simulink model "Battery_Management_System"  (R2025b)
settings: Solver=ode1be  StartTime=0.0  StopTime=600  FixedStep=0.1  MaxStep=0.05  RelTol=1e-3  AbsTol=1e-3
PreLoadFcn:
  | Battery_Management_System_param
undefined symbols (not defined in the file): AH, ambient, coolantTemp, iniSOC1, R0_mat, R12, R1_mat, samplingTime, SOC_vec, T_vec, Tau1_mat, V0_mat
libraries: nesl_utility x12, fl_lib x6, ee_lib x2, batteryModule_lib x2
Description:
  | Battery Management System
  | 
  | Copyright 2021-2025 The MathWorks, Inc.
settings Model: Creator=vikrants  LastModifiedBy=smiller
settings SolverCC: AutoScaleAbsTol=off  AlgebraicLoopSolver=TrustRegion
settings DataIOCC: ReturnWorkspaceOutputs=off  SignalLoggingName=logsout_Battery_Pack_Thermal_Management
settings OptimizationCC: ReuseModelBlockBuffer=off
settings DebuggingCC: UnconnectedInputMsg=warning  UnconnectedOutputMsg=warning  UnconnectedLineMsg=warning  SymbolicDimsDataTypeCodeGenerationDiagnostic=none
settings ModelReferenceCC: EnableRefExpFcnMdlSchedulingChecks=on
settings SFSimCC: CustomCodeUndefinedFunction=UseInterfaceOnly
settings RTWCC: GPUComputeCapability=3.5  DLArmComputeVersion=19.05
settings SimscapeCC: SimscapeLogType=all  SimscapeLogSimulationStatistics=on  SimscapeLogName=simlog_Battery_Management_System  SimscapeLogDataHistory=250000.0

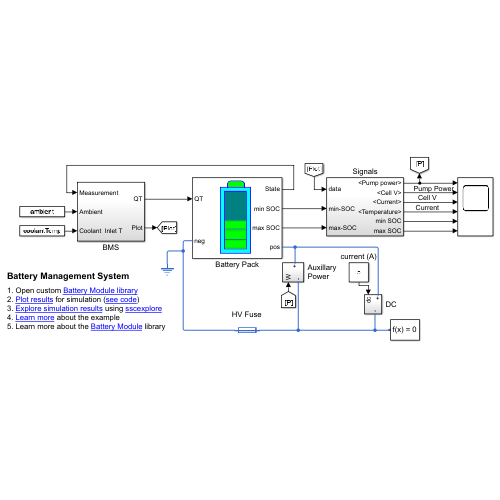
[thumbnail: Simulink's stored preview of the top-level diagram]
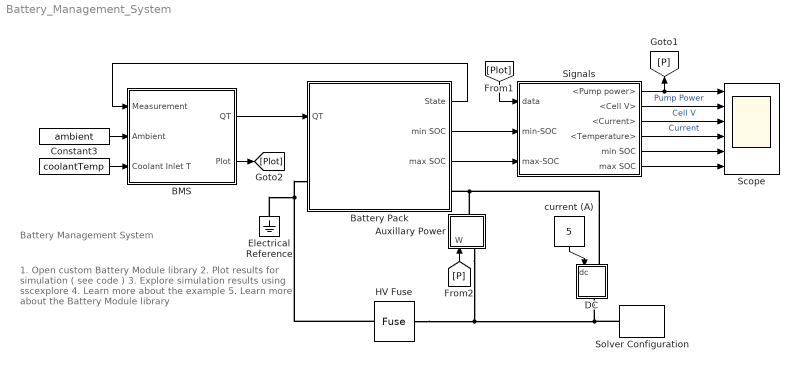
== system Battery_Management_System ==
  note: 1. Open custom Battery Module library
      | 2. Plot results for simulation ( see code )
      | 3. Explore simulation results using sscexplore
      | 4. Learn more about the example
      | 5. Learn more about the Battery Module library
  note: Battery Management System
  " " : Constant  Value=coolantTemp  SampleTime=samplingTime
  Auxillary Power : Subsystem
  BMS : Subsystem
  Battery Pack : Subsystem
      mask Display: image('Battery_Management_System_icon.png'); % Use "Edit Image" on toolstrip to change.
  Constant3 : Constant  Value=ambient  SampleTime=samplingTime
  DC : Subsystem
  Electrical Reference : fl_lib/Electrical/Electrical Elements/Electrical Reference
  HV Fuse : ee_lib/Switches & Breakers/Fuse  prm=1  I_rated=100 A  melt_margin=4  T_fuse=0 s  I2t=1 s*A^2  I_vec=[1.9, 2, 2.5, 30] A  t_vec=[10000, 1, .3, .001] s  R_closed=0.0005 Ohm  G_open=1e-8 1/Ohm  exposemeasurement=ee.enum.exposemeasurement.hidden
      settings: InternalSimscapePortConfiguration="{\"Bottom\":[],\"Left\":[{\"id\":\"p\",\"label\":\"\",\"type\":\"foundation.electrical.electrical\"}],\"Right\":[{\"id\":\"n\",\"label\":\"\",\"type\":\"foundation.electrical.electrical\"}],\"Top\":[]}"
  Scope : Scope  NumInputPorts=6
      settings: ActiveDisplayYMinimum=-15.625  ActiveDisplayYMaximum=140.625  DataLoggingVariableName=Battery_Management_System_Scope
  Signals : Subsystem
  Solver Configuration : nesl_utility/Solver Configuration  PhysicalDomain=network_engine_domain  SubClassName=solver  LeftPortType=input  RightPortType=generic  Tones=[]  Harmonics=[]  SimulateNoise=off  Profile=off  UseLocalSampling=off  EnableSwitchedLinearOptims=on  FrequencyDomain=off  UseCCode=off  RelTol=0.001  AbsTol=1e-06  MinStep=1e-09  ToWorkspace=off  RevertToSquareIcSolve=off  NumHomotopyIterations=100  PhasorMode=off  PhasorModeNumHarmonics=1  ConsistencySolver=NEWTON_FTOL  IndexReductionMethod=DerivativeReplacement  DoDC=off  ResidualTolerance=1e-09  ConsistencyTolSource=GLOBAL  ConsistencyAbsTol=0.001  ConsistencyRelTol=0.001  ConsistencyTolFactor=0.001  UseLocalSolver=on  LocalSolverChoice=NE_BACKWARD_EULER_ADVANCER  ResolveIndetEquations=on  FunctionEvalNumThread=1  LocalSolverSampleTime=0.1  DoFixedCost=on  MaxNonlinIter=3  MaxModeIter=2  ComputeImpulses=off  ImpulseIterations=2  LinearAlgebra=auto  LinearAlgebraNumThread=0  EquationFormulation=NE_TIME_EF  DelaysMemoryBudget=1024  AutomaticFiltering=on  FilteringTimeConstant=0.001  PartitionStorageMethod=AS_NEEDED  PartitionMemoryBudget=1024  PartitionMethod=ROBUST  MultibodyUseLocalSolver=off  MultibodyLocalSolverChoice=ODE1  MultibodyLocalSolverSampleTime=0.001
  current (A) : Constant  Value=5
  wires:
  Battery Pack/1(State) -> BMS/1(Measurement)
  Constant3/1 -> BMS/2(Ambient)
  " "/1 -> BMS/3(Coolant Inlet T)
  BMS/1(QT) -> Battery Pack/1(QT)
  BMS/2(Plot) -> [Plot]
  [P] -> Auxillary Power/1(W)
  current (A)/1 -> DC/1(dc)
  Battery Pack/3(max SOC) -> Signals/3(max-SOC)
  Signals/1(<Pump power>) -> Scope/1, [P]  "Pump Power"
  [Plot] -> Signals/1(data)
  Battery Pack/2(min SOC) -> Signals/2(min-SOC)
  Signals/2(<Cell V>) -> Scope/2  "Cell V"
  Signals/3(<Current>) -> Scope/3  "Current"
  Signals/4(<Temperature>) -> Scope/4
  Signals/5(min SOC) -> Scope/5
  Signals/6(max SOC) -> Scope/6
  connections:
  Auxillary Power/LConn1 -- HV Fuse/LConn1 -- Solver Configuration/RConn1 -- DC/RConn1
  Auxillary Power/RConn1 -- Battery Pack/RConn1 -- DC/LConn1
  HV Fuse/RConn1 -- Electrical Reference/LConn1 -- Battery Pack/LConn1

== system Battery_Management_System/Auxillary Power ==
  W : Inport
  Aux. Power : ee_lib/Passive/Dynamic Load  load_type=ee.enum.dc_ac.dc  min_supply_voltage=20 V  pow_min=1e-3 W  G_reverse=1e-6 S  deltaV=1e-3 V  f0=60 Hz  Vrms_min=200 V  tau=0.01 s  Vrms_ini=300 V  Vang_ini=0 deg
      settings: InternalSimscapePortConfiguration="{\"Bottom\":[],\"Left\":[{\"id\":\"p\",\"label\":\"+\",\"type\":\"foundation.electrical.electrical\"}],\"Right\":[{\"id\":\"n\",\"label\":\"-\",\"type\":\"foundation.electrical.electrical\"}],\"Top\":[{\"id\":\"P\",\"label\":\"P\",\"type\":\"input\"}]}"
  P : nesl_utility/Simulink-PS Converter  PhysicalDomain=network_engine_domain  SubClassName=ps_input  LeftPortType=input  RightPortType=output  PseudoPeriodic=off  Frequencies=[]  NoiseDistribution=none  NoiseParameters=[]  Unit=J/s  AffineConversion=off  FilteringAndDerivatives=provide  SimscapeFilterOrder=1  InputFilterTimeConstant=0.001  UdotUserProvided=0
  + : PMIOPort  Side=Right
  - : PMIOPort  Port=2  Side=Left
  wires:
  W/1 -> P/1
  connections:
  P/RConn1 -- Aux. Power/LConn2
  Aux. Power/LConn1 -- -/RConn1
  Aux. Power/RConn1 -- +/RConn1

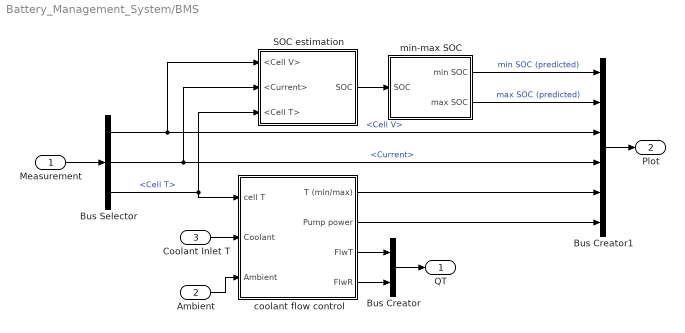
== system Battery_Management_System/BMS ==
  Measurement : Inport
  Ambient : Inport  Port=2  Unit=K
  Coolant Inlet T : Inport  Port=3  Unit=K
  Bus Creator : BusCreator  Inputs=2
  Bus Creator1 : BusCreator  Inputs=6
  Bus Selector : BusSelector  OutputSignals=Cell V,Current,Cell T
  SOC estimation : Subsystem
  coolant flow control : Subsystem
  min-max SOC : Subsystem
  QT : Outport
  Plot : Outport  Port=2
  wires:
  Bus Creator/1 -> QT/1
  Measurement/1 -> Bus Selector/1
  Bus Creator1/1 -> Plot/1
  Bus Selector/1 -> SOC estimation/1(<Cell V>), Bus Creator1/3  "<Cell V>"
  Bus Selector/3 -> SOC estimation/3(<Cell T>), coolant flow control/1(cell T)  "<Cell T>"
  Bus Selector/2 -> Bus Creator1/4, SOC estimation/2(<Current>)  "<Current>"
  SOC estimation/1(SOC) -> min-max SOC/1(SOC)
  min-max SOC/1(min SOC) -> Bus Creator1/1  "min SOC (predicted)"
  min-max SOC/2(max SOC) -> Bus Creator1/2  "max SOC (predicted)"
  Coolant Inlet T/1 -> coolant flow control/2(Coolant)
  Ambient/1 -> coolant flow control/3(Ambient)
  coolant flow control/3(FlwT) -> Bus Creator/1
  coolant flow control/4(FlwR) -> Bus Creator/2
  coolant flow control/2(Pump power) -> Bus Creator1/6
  coolant flow control/1(T (min/max)) -> Bus Creator1/5

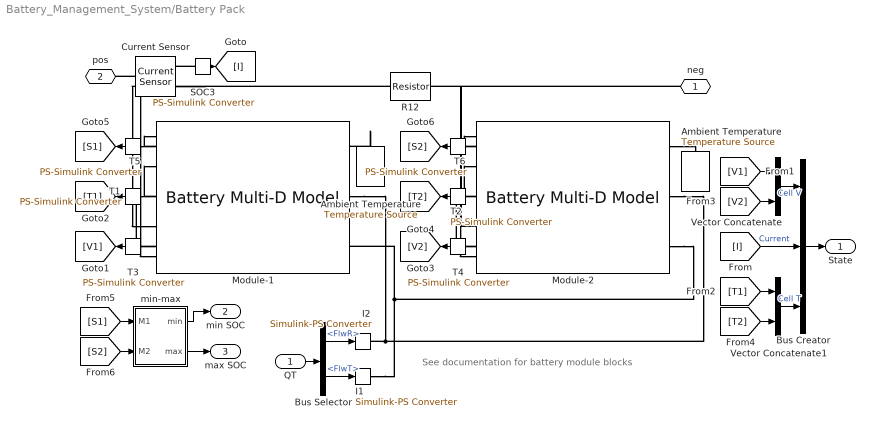
== system Battery_Management_System/Battery Pack ==
  note: See documentation for battery module blocks
  QT : Inport
  Ambient Temperature : fl_lib/Thermal/Thermal Sources/Temperature Source  temperature=ambient K
  "Ambient Temperature " : fl_lib/Thermal/Thermal Sources/Temperature Source  temperature=ambient K
  Bus Creator : BusCreator  Inputs=3
  Bus Selector : BusSelector  OutputSignals=FlwR,FlwT
  Current Sensor : fl_lib/Electrical/Electrical Sensors/Current Sensor
  I1 : nesl_utility/Simulink-PS Converter  PhysicalDomain=network_engine_domain  SubClassName=ps_input  LeftPortType=input  RightPortType=output  PseudoPeriodic=off  Frequencies=[]  NoiseDistribution=none  NoiseParameters=[]  Unit=K  AffineConversion=off  FilteringAndDerivatives=provide  SimscapeFilterOrder=1  InputFilterTimeConstant=0.001  UdotUserProvided=0
  I2 : nesl_utility/Simulink-PS Converter  PhysicalDomain=network_engine_domain  SubClassName=ps_input  LeftPortType=input  RightPortType=output  PseudoPeriodic=off  Frequencies=[]  NoiseDistribution=none  NoiseParameters=[]  Unit=1  AffineConversion=off  FilteringAndDerivatives=provide  SimscapeFilterOrder=1  InputFilterTimeConstant=0.001  UdotUserProvided=0
  Module-1 : batteryModule_lib/Battery Multi-D Model  modelComplexity=batteryModule.batteryAbstractionLevel.detailed  LUTpointsTemp=T_vec K  cellAH=AH A*hr  LUTpointsSOC=SOC_vec  V0_mat=V0_mat V  prm_dir=simscape.enum.tablebattery.prm_dir.noCurrentDirectionality  R0_mat=R0_mat Ohm  R0_dis_mat=[.03, .015, .002; .04, .017, .008; .039, .012, .006; .027, .013, .021] Ohm  R0_ch_mat=[.03, .015, .002; .04, .017, .008; .039, .012, .006; .027, .013, .021] Ohm  prm_leak=simscape.enum.tablebattery.prm_leak.disabled  Rleak_vec=[8000, 7000, 6000] Ohm  extrapolation_option=simscape.enum.extrapolation.linear  prm_dyn=simscape.enum.tablebattery.prm_dyn.rc1  R1_mat=R1_mat Ohm  tau1_mat=Tau1_mat s  R2_mat=R2_mat Ohm  tau2_mat=Tau2_mat s  R3_mat=[.014, .382, .407; .028, .006, .007; .014, .007, .006; .333, .956, .912] Ohm  tau3_mat=[1, 44, 5644; 11, 24, 506; 2, 14, 330; 3310, 13419, 30216] s  R4_mat=[.014, .382, .407; .028, .006, .007; .014, .007, .006; .333, .956, .912] Ohm  tau4_mat=[1, 44, 5644; 11, 24, 506; 2, 14, 330; 3310, 13419, 30216] s  R5_mat=[.014, .382, .407; .028, .006, .007; .014, .007, .006; .333, .956, .912] Ohm  tau5_mat=[1, 44, 5644; 11, 24, 506; 2, 14, 330; 3310, 13419, 30216] s  prm_fade=simscape.enum.tablebattery.prm_fade.equations  N0=Ndisc  dV0=delV0  dR0=delR0  dAH=delAH0  dRleak=0  dR1=delR1  dR2=delR2  dR3=0  dR4=0  dR5=0  N0vec=[100, 200, 300]  Tfadevec=[298.15, 323.15] K  dV0vec=[0, 0, 0]  dR0vec=[0, 0, 0]  dAHvec=[0, 0, 0]  dRleakvec=[0, 0, 0]  dR1vec=[0, 0, 0]  dR2vec=[0, 0, 0]  dR3vec=[0, 0, 0]  dR4vec=[0, 0, 0]  dR5vec=[0, 0, 0]  dV0mat=[0, 0; 0, 0; 0, 0]  dR0mat=[0, 0; 0, 0; 0, 0]  dAHmat=[0, 0; 0, 0; 0, 0]  dRleakmat=[0, 0; 0, 0; 0, 0]  dR1mat=[0, 0; 0, 0; 0, 0]  dR2mat=[0, 0; 0, 0; 0, 0]  dR3mat=[0, 0; 0, 0; 0, 0]  dR4mat=[0, 0; 0, 0; 0, 0]  dR5mat=[0, 0; 0, 0; 0, 0]  cellThermalMass=MdotCp J/K  cellThermalCond=K_cell W/(m*K)  cellThermalCond_inPlane=20 W/(m*K)  Ns=Ns1  Np=Np1  cellTypeSelection=batteryModule.batteryTypeSelection.pouch  cellHeight=cell_H m  cellWidth=cell_W m  cellThickness=cell_T m  cellDiameter=0.018 m  cellCylinLine=3  moduleExternalR=Rext1 Ohm  moduleCellBalancing=batteryModule.batteryCellBalancing.none  passiveShuntR=50 Ohm  passiveSWclosedR=0.01 Ohm  passiveSWopenCond=1e-8 1/Ohm  passiveSWthreshold=0.5  moduleCellVoltages=batteryModule.batteryCellVoltages.yes  thermalManagement=batteryModule.batteryCoolingSystem.thermalPort  cellHeatTrCoeff=h_cell W/(m^2 * K)  thermal_moduleBottom=batteryModule.batteryThermalPortSelection.thermalLUT  htc_bottom=1 W/(m^2 * K)  moduleCooling_b=Q1 W/K  LUTpointsFlowrate_b=Flowrate_vec kg/s  LUTpointsTemp_b=T_vec K  thermal_moduleTop=batteryModule.batteryThermalPortSelection.convectionBC  htc_top=h_cell W/(m^2 * K)  moduleCooling_t=zeros(3, 6, 10) W/K  LUTpointsFlowrate_t=[.01, .02, .03, .04, .05, .06] kg/s  LUTpointsTemp_t=[273.15, 298.15, 323.15] K  thermal_moduleRight=batteryModule.batteryThermalPortSelection.convectionBC  htc_right=h_cell W/(m^2 * K)  moduleCooling_r=zeros(3, 6, 10) W/K  LUTpointsFlowrate_r=[.01, .02, .03, .04, .05, .06] kg/s  LUTpointsTemp_r=[273.15, 298.15, 323.15] K  thermal_moduleLeft=batteryModule.batteryThermalPortSelection.convectionBC  htc_left=h_cell W/(m^2 * K)  moduleCooling_l=zeros(3, 6, 10) W/K  LUTpointsFlowrate_l=[.01, .02, .03, .04, .05, .06] kg/s  LUTpointsTemp_l=[273.15, 298.15, 323.15] K  thermal_modulePos=batteryModule.batteryThermalPortSelection.convectionBC  htc_pos=h_cell W/(m^2 * K)  moduleCooling_p=zeros(3, 6, 10) W/K  LUTpointsFlowrate_p=[.01, .02, .03, .04, .05, .06] kg/s  LUTpointsTemp_p=[273.15, 298.15, 323.15] K  thermal_moduleNeg=batteryModule.batteryThermalPortSelection.convectionBC  htc_neg=h_cell W/(m^2 * K)  moduleCooling_n=zeros(3, 6, 10) W/K  LUTpointsFlowrate_n=[.01, .02, .03, .04, .05, .06] kg/s  LUTpointsTemp_n=[273.15, 298.15, 323.15] K  moduleExtHeat=extQ1 W  cellTemp=iniT1 K  cellSOC=iniSOC1  moduleCellAHpercentVar=iniAH1  moduleCellLeakPercentVar=ones(1, 10)  moduleCellR0PercentVar=iniR01
      settings: InternalSimscapePortConfiguration="{\"Bottom\":[],\"Left\":[{\"id\":\"outputCellSOC\",\"label\":\"SOC\",\"type\":\"output\"},{\"id\":\"outputCellTemp\",\"label\":\"Temp\",\"type\":\"output\"},{\"id\":\"outputCellV\",\"label\":\"V\",\"type\":\"output\"}],\"Right\":[{\"id\":\"H\",\"label\":\"Amb\",\"type\":\"foundation.thermal.thermal\"},{\"id\":\"frac_b\",\"label\":\"FlwR\",\"type\":\"input\"},{\"id\":\"delT_b\",\"label\":\"FlwT\",\"type\":\"input\"}],\"Top\":[{\"id\":\"p\",\"label\":\"pos\",\"type\":\"foundation.electrical.electrical\"},{\"id\":\"n\",\"label\":\"neg\",\"type\":\"foundation.electrical.electrical\"}]}"
  Module-2 : batteryModule_lib/Battery Multi-D Model  modelComplexity=batteryModule.batteryAbstractionLevel.detailed  LUTpointsTemp=T_vec K  cellAH=AH A*hr  LUTpointsSOC=SOC_vec  V0_mat=V0_mat V  prm_dir=simscape.enum.tablebattery.prm_dir.noCurrentDirectionality  R0_mat=R0_mat Ohm  R0_dis_mat=[.03, .015, .002; .04, .017, .008; .039, .012, .006; .027, .013, .021] Ohm  R0_ch_mat=[.03, .015, .002; .04, .017, .008; .039, .012, .006; .027, .013, .021] Ohm  prm_leak=simscape.enum.tablebattery.prm_leak.disabled  Rleak_vec=[8000, 7000, 6000] Ohm  extrapolation_option=simscape.enum.extrapolation.linear  prm_dyn=simscape.enum.tablebattery.prm_dyn.rc1  R1_mat=R1_mat Ohm  tau1_mat=Tau1_mat s  R2_mat=R2_mat Ohm  tau2_mat=Tau2_mat s  R3_mat=[.014, .382, .407; .028, .006, .007; .014, .007, .006; .333, .956, .912] Ohm  tau3_mat=[1, 44, 5644; 11, 24, 506; 2, 14, 330; 3310, 13419, 30216] s  R4_mat=[.014, .382, .407; .028, .006, .007; .014, .007, .006; .333, .956, .912] Ohm  tau4_mat=[1, 44, 5644; 11, 24, 506; 2, 14, 330; 3310, 13419, 30216] s  R5_mat=[.014, .382, .407; .028, .006, .007; .014, .007, .006; .333, .956, .912] Ohm  tau5_mat=[1, 44, 5644; 11, 24, 506; 2, 14, 330; 3310, 13419, 30216] s  prm_fade=simscape.enum.tablebattery.prm_fade.equations  N0=Ndisc  dV0=delV0  dR0=delR0  dAH=delAH0  dRleak=0  dR1=delR1  dR2=delR2  dR3=0  dR4=0  dR5=0  N0vec=[100, 200, 300]  Tfadevec=[298.15, 323.15] K  dV0vec=[0, 0, 0]  dR0vec=[0, 0, 0]  dAHvec=[0, 0, 0]  dRleakvec=[0, 0, 0]  dR1vec=[0, 0, 0]  dR2vec=[0, 0, 0]  dR3vec=[0, 0, 0]  dR4vec=[0, 0, 0]  dR5vec=[0, 0, 0]  dV0mat=[0, 0; 0, 0; 0, 0]  dR0mat=[0, 0; 0, 0; 0, 0]  dAHmat=[0, 0; 0, 0; 0, 0]  dRleakmat=[0, 0; 0, 0; 0, 0]  dR1mat=[0, 0; 0, 0; 0, 0]  dR2mat=[0, 0; 0, 0; 0, 0]  dR3mat=[0, 0; 0, 0; 0, 0]  dR4mat=[0, 0; 0, 0; 0, 0]  dR5mat=[0, 0; 0, 0; 0, 0]  cellThermalMass=MdotCp J/K  cellThermalCond=K_cell W/(m*K)  cellThermalCond_inPlane=20 W/(m*K)  Ns=Ns2  Np=Np2  cellTypeSelection=batteryModule.batteryTypeSelection.pouch  cellHeight=cell_H m  cellWidth=cell_W m  cellThickness=cell_T m  cellDiameter=0.018 m  cellCylinLine=3  moduleExternalR=Rext2 Ohm  moduleCellBalancing=batteryModule.batteryCellBalancing.none  passiveShuntR=50 Ohm  passiveSWclosedR=0.01 Ohm  passiveSWopenCond=1e-8 1/Ohm  passiveSWthreshold=0.5  moduleCellVoltages=batteryModule.batteryCellVoltages.yes  thermalManagement=batteryModule.batteryCoolingSystem.thermalPort  cellHeatTrCoeff=h_cell W/(m^2 * K)  thermal_moduleBottom=batteryModule.batteryThermalPortSelection.thermalLUT  htc_bottom=1 W/(m^2 * K)  moduleCooling_b=Q2 W/K  LUTpointsFlowrate_b=Flowrate_vec kg/s  LUTpointsTemp_b=T_vec K  thermal_moduleTop=batteryModule.batteryThermalPortSelection.convectionBC  htc_top=h_cell W/(m^2 * K)  moduleCooling_t=zeros(3, 6, 10) W/K  LUTpointsFlowrate_t=[.01, .02, .03, .04, .05, .06] kg/s  LUTpointsTemp_t=[273.15, 298.15, 323.15] K  thermal_moduleRight=batteryModule.batteryThermalPortSelection.convectionBC  htc_right=h_cell W/(m^2 * K)  moduleCooling_r=zeros(3, 6, 10) W/K  LUTpointsFlowrate_r=[.01, .02, .03, .04, .05, .06] kg/s  LUTpointsTemp_r=[273.15, 298.15, 323.15] K  thermal_moduleLeft=batteryModule.batteryThermalPortSelection.convectionBC  htc_left=h_cell W/(m^2 * K)  moduleCooling_l=zeros(3, 6, 10) W/K  LUTpointsFlowrate_l=[.01, .02, .03, .04, .05, .06] kg/s  LUTpointsTemp_l=[273.15, 298.15, 323.15] K  thermal_modulePos=batteryModule.batteryThermalPortSelection.convectionBC  htc_pos=h_cell W/(m^2 * K)  moduleCooling_p=zeros(3, 6, 10) W/K  LUTpointsFlowrate_p=[.01, .02, .03, .04, .05, .06] kg/s  LUTpointsTemp_p=[273.15, 298.15, 323.15] K  thermal_moduleNeg=batteryModule.batteryThermalPortSelection.convectionBC  htc_neg=h_cell W/(m^2 * K)  moduleCooling_n=zeros(3, 6, 10) W/K  LUTpointsFlowrate_n=[.01, .02, .03, .04, .05, .06] kg/s  LUTpointsTemp_n=[273.15, 298.15, 323.15] K  moduleExtHeat=extQ2 W  cellTemp=iniT2 K  cellSOC=iniSOC2  moduleCellAHpercentVar=iniAH2  moduleCellLeakPercentVar=ones(1, 10)  moduleCellR0PercentVar=iniR02
      settings: InternalSimscapePortConfiguration="{\"Bottom\":[],\"Left\":[{\"id\":\"outputCellSOC\",\"label\":\"SOC\",\"type\":\"output\"},{\"id\":\"outputCellTemp\",\"label\":\"Temp\",\"type\":\"output\"},{\"id\":\"outputCellV\",\"label\":\"V\",\"type\":\"output\"}],\"Right\":[{\"id\":\"H\",\"label\":\"Amb\",\"type\":\"foundation.thermal.thermal\"},{\"id\":\"frac_b\",\"label\":\"FlwR\",\"type\":\"input\"},{\"id\":\"delT_b\",\"label\":\"FlwT\",\"type\":\"input\"}],\"Top\":[{\"id\":\"p\",\"label\":\"pos\",\"type\":\"foundation.electrical.electrical\"},{\"id\":\"n\",\"label\":\"neg\",\"type\":\"foundation.electrical.electrical\"}]}"
  R12 : fl_lib/Electrical/Electrical Elements/Resistor  R=R12 Ohm  i_specify=off  i_priority=None  i=0 A  i_nominal_specify=off  i_nominal_value=1  i_nominal_unit=A  v_specify=off  v_priority=None  v=0 V  v_nominal_specify=off  v_nominal_value=1  v_nominal_unit=V
  SOC3 : nesl_utility/PS-Simulink Converter  PhysicalDomain=network_engine_domain  SubClassName=ps_output  LeftPortType=input  RightPortType=output  PseudoPeriodic=off  Frequencies=[]  VectorFormat=1-D array  Unit=inherit  AffineConversion=off
  T{1..6} (6 alike) : nesl_utility/PS-Simulink Converter  PhysicalDomain=network_engine_domain  SubClassName=ps_output  LeftPortType=input  RightPortType=output  PseudoPeriodic=off  Frequencies=[]  VectorFormat=1-D array  Unit=inherit  AffineConversion=off
  Vector Concatenate : Concatenate
  Vector Concatenate1 : Concatenate
  min-max : Subsystem
  neg : PMIOPort  Side=Left
  pos : PMIOPort  Port=2  Side=Right
  State : Outport
  min SOC : Outport  Port=2
  max SOC : Outport  Port=3
  wires:
  Bus Creator/1 -> State/1
  Vector Concatenate/1 -> Bus Creator/1  "Cell V"
  SOC3/1 -> [I]
  [V1] -> Vector Concatenate/1
  T3/1 -> [V1]
  [T1] -> Vector Concatenate1/1
  T2/1 -> [T2]
  T4/1 -> [V2]
  T1/1 -> [T1]
  [T2] -> Vector Concatenate1/2
  [V2] -> Vector Concatenate/2
  Vector Concatenate1/1 -> Bus Creator/3  "Cell T"
  [I] -> Bus Creator/2  "Current"
  QT/1 -> Bus Selector/1
  Bus Selector/1 -> I2/1  "<FlwR>"
  Bus Selector/2 -> I1/1  "<FlwT>"
  T5/1 -> [S1]
  T6/1 -> [S2]
  min-max/1(min) -> min SOC/1
  min-max/2(max) -> max SOC/1
  [S1] -> min-max/1(M1)
  [S2] -> min-max/2(M2)
  connections:
  T1/LConn1 -- Module-1/LConn2
  R12/LConn1 -- Module-1/LConn5
  T2/LConn1 -- Module-2/LConn2
  Module-2/LConn4 -- R12/RConn1
  neg/RConn1 -- Module-2/LConn5
  T3/LConn1 -- Module-1/LConn3
  T4/LConn1 -- Module-2/LConn3
  Current Sensor/LConn1 -- pos/RConn1
  Current Sensor/RConn2 -- Module-1/LConn4
  SOC3/LConn1 -- Current Sensor/RConn1
  Ambient Temperature/LConn1 -- Module-1/RConn1
  Module-2/RConn1 -- "Ambient Temperature "/LConn1
  Module-1/RConn2 -- Module-2/RConn2 -- I2/RConn1
  I1/RConn1 -- Module-2/RConn3 -- Module-1/RConn3
  T5/LConn1 -- Module-1/LConn1
  T6/LConn1 -- Module-2/LConn1

== system Battery_Management_System/DC ==
  dc : Inport
  Current Source : fl_lib/Electrical/Electrical Sources/Controlled Current Source
  Gain : Gain  Gain=-1
  I : nesl_utility/Simulink-PS Converter  PhysicalDomain=network_engine_domain  SubClassName=ps_input  LeftPortType=input  RightPortType=output  PseudoPeriodic=off  Frequencies=[]  NoiseDistribution=none  NoiseParameters=[]  Unit=A  AffineConversion=off  FilteringAndDerivatives=provide  SimscapeFilterOrder=1  InputFilterTimeConstant=0.001  UdotUserProvided=0
  + : PMIOPort  Side=Left
  - : PMIOPort  Port=2  Side=Right
  wires:
  Gain/1 -> I/1
  dc/1 -> Gain/1
  connections:
  I/RConn1 -- Current Source/RConn1
  Current Source/LConn1 -- +/RConn1
  Current Source/RConn2 -- -/RConn1

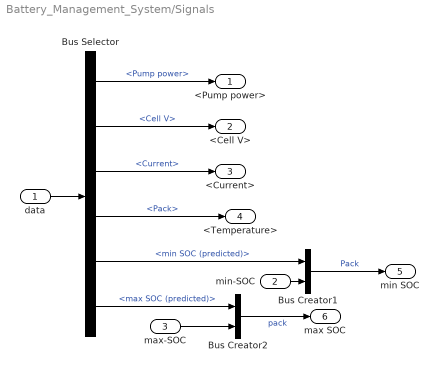
== system Battery_Management_System/Signals ==
  data : Inport
  min-SOC : Inport  Port=2
  max-SOC : Inport  Port=3
  Bus Creator1 : BusCreator  Inputs=2
  Bus Creator2 : BusCreator  Inputs=2
  Bus Selector : BusSelector  OutputSignals=Pump power,Cell V,Current,Pack,min SOC (predicted),max SOC (predicted)
  <Pump power> : Outport
  <Cell V> : Outport  Port=2
  <Current> : Outport  Port=3
  <Temperature> : Outport  Port=4
  min SOC : Outport  Port=5
  max SOC : Outport  Port=6
  wires:
  min-SOC/1 -> Bus Creator1/2
  Bus Creator2/1 -> max SOC/1  "pack"
  Bus Selector/2 -> <Cell V>/1  "<Cell V>"
  Bus Creator1/1 -> min SOC/1  "Pack"
  max-SOC/1 -> Bus Creator2/2
  Bus Selector/4 -> <Temperature>/1  "<Pack>"
  data/1 -> Bus Selector/1
  Bus Selector/5 -> Bus Creator1/1  "<min SOC (predicted)>"
  Bus Selector/3 -> <Current>/1  "<Current>"
  Bus Selector/1 -> <Pump power>/1  "<Pump power>"
  Bus Selector/6 -> Bus Creator2/1  "<max SOC (predicted)>"

== system Battery_Management_System/BMS/SOC estimation ==
  <Cell V> : Inport
  <Current> : Inport  Port=2
  <Cell T> : Inport  Port=3
  AEKF 1TC : Subsystem  TreatAsAtomicUnit=on
  SeriesStringData <Ns=20,Np=1> : MATLAB Function  TreatAsAtomicUnit=on
  SOC : Outport
  wires:
  SeriesStringData <Ns=20,Np=1>/1(Is) -> AEKF 1TC/1(Current)
  <Cell V>/1 -> SeriesStringData <Ns=20,Np=1>/3(V)
  AEKF 1TC/1(SOC) -> SOC/1
  SeriesStringData <Ns=20,Np=1>/3(Vs) -> AEKF 1TC/3(Voltage)
  <Current>/1 -> SeriesStringData <Ns=20,Np=1>/1(I)
  SeriesStringData <Ns=20,Np=1>/2(Ts) -> AEKF 1TC/2(Temperature)
  <Cell T>/1 -> SeriesStringData <Ns=20,Np=1>/2(T)

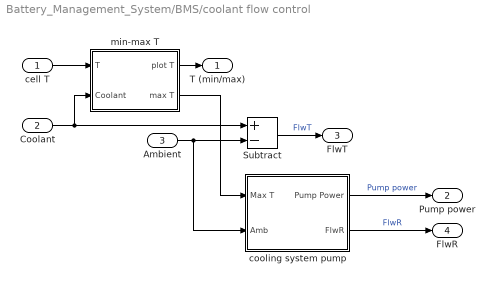
== system Battery_Management_System/BMS/coolant flow control ==
  cell T : Inport
  Coolant : Inport  Port=2
  Ambient : Inport  Port=3
  Subtract : Sum  Inputs=+-
  cooling system pump : Subsystem
  min-max T : Subsystem
  T (min/max) : Outport
  Pump power : Outport  Port=2
  FlwT : Outport  Port=3
  FlwR : Outport  Port=4
  wires:
  cell T/1 -> min-max T/1(T)
  min-max T/2(max T) -> cooling system pump/1(Max T)
  Coolant/1 -> min-max T/2(Coolant), Subtract/1
  cooling system pump/2(FlwR) -> FlwR/1  "FlwR"
  cooling system pump/1(Pump Power) -> Pump power/1  "Pump power"
  Subtract/1 -> FlwT/1  "FlwT"
  min-max T/1(plot T) -> T (min/max)/1
  Ambient/1 -> cooling system pump/2(Amb), Subtract/2

== system Battery_Management_System/BMS/min-max SOC ==
  SOC : Inport
  MinMax2 : MinMax
  MinMax3 : MinMax  Function=max
  min SOC : Outport
  max SOC : Outport  Port=2
  wires:
  MinMax3/1 -> max SOC/1
  SOC/1 -> MinMax2/1, MinMax3/1
  MinMax2/1 -> min SOC/1

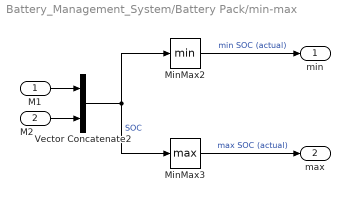
== system Battery_Management_System/Battery Pack/min-max ==
  M1 : Inport
  M2 : Inport  Port=2
  MinMax2 : MinMax
  MinMax3 : MinMax  Function=max
  Vector Concatenate2 : Concatenate
  min : Outport
  max : Outport  Port=2
  wires:
  MinMax3/1 -> max/1  "max SOC (actual)"
  MinMax2/1 -> min/1  "min SOC (actual)"
  Vector Concatenate2/1 -> MinMax3/1, MinMax2/1  "SOC"
  M1/1 -> Vector Concatenate2/1
  M2/1 -> Vector Concatenate2/2

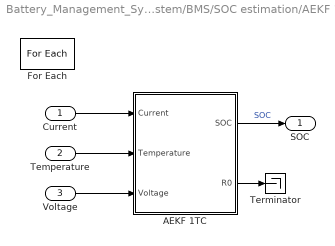
== system Battery_Management_System/BMS/SOC estimation/AEKF 1TC ==
  Current : Inport  Partition=on  PartitionDimension=1  PartitionWidth=1  PartitionOffset=0
  Temperature : Inport  Port=2  Partition=on  PartitionDimension=1  PartitionWidth=1  PartitionOffset=0
  Voltage : Inport  Port=3  Partition=on  PartitionDimension=1  PartitionWidth=1  PartitionOffset=0
  AEKF 1TC : Subsystem  mask(Adaptive Extended Kalman Filter SOC estimator){SOC_vec=SOC_vec, T_vec=T_vec, R0_mat=R0_mat, R1_mat=R1_mat, tau1_mat=Tau1_mat, V0_mat=V0_mat, AH=AH, Reol=0.05, Ts=1, Q=1e-8*eye(3), R=1e-2, P0=[1e-5 0 0; 0 1 0; 0 0 0.0125], x0=[iniSOC1(1);0;9.4e-3]}
      mask prompts: SOC_vec "Vector of state-of-charge values, SOC"; T_vec "Vector of temperatures, T"; R0_mat "Terminal resistance, R0(SOC,T)"; R1_mat "First polarization resistance, R1(SOC,T)"; tau1_mat "First time constant, tau1(SOC,T)"; V0_mat "No-load voltage, V0(SOC,T)"; AH "Ampere-hour rating"; Reol "End of life resistance"; Ts "Sample time"; Q "Covariance of the process noise, Q"; R "Covariance matrix of the measurement noise, R"; P0 "Initial state error covariance, P0"; x0 "Initial state"
      mask help: This block implements an Adaptive Extended Kalman Filter battery SOC estimator based on a one time constant battery model.
      mask init:
      | C1_mat=tau1_mat./R1_mat;
      | 
      | dV0_mat=zeros(size(V0_mat));
      | [n_soc,m_soc]=size(SOC_vec);
      | if n_soc<m_soc
      |     dV0_mat(2:end,:)=diff(V0_mat,1,1)./diff(SOC_vec');
      | else
      |     dV0_mat(2:end,:)=diff(V0_mat,1,1)./diff(SOC_vec);
      | end
      mask DialogControl Container7 Prompt: System Model
      mask DialogControl Container10 Prompt: Kalman Filter
  For Each : ForEach  DisableCoverage=on
  Terminator : Terminator
  SOC : Outport  ConcatenationDimension=1
  wires:
  Current/1 -> AEKF 1TC/1(Current)
  AEKF 1TC/1(SOC) -> SOC/1  "SOC"
  Temperature/1 -> AEKF 1TC/2(Temperature)
  Voltage/1 -> AEKF 1TC/3(Voltage)
  AEKF 1TC/2(R0) -> Terminator/1

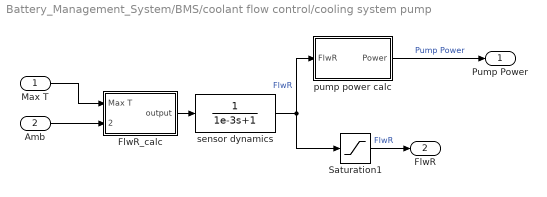
== system Battery_Management_System/BMS/coolant flow control/cooling system pump ==
  Max T : Inport
  Amb : Inport  Port=2
  FlwR_calc : Subsystem
  Saturation1 : Saturate  UpperLimit=1  LowerLimit=0.01
  pump power calc : Subsystem
  sensor dynamics : TransferFcn  Denominator=[1e-3 1]
  Pump Power : Outport
  FlwR : Outport  Port=2
  wires:
  sensor dynamics/1 -> Saturation1/1, pump power calc/1(FlwR)  "FlwR"
  Amb/1 -> FlwR_calc/2(Ambient)
  Max T/1 -> FlwR_calc/1(Max T)
  pump power calc/1(Power) -> Pump Power/1  "Pump Power"
  FlwR_calc/1(output) -> sensor dynamics/1
  Saturation1/1 -> FlwR/1  "FlwR"

== system Battery_Management_System/BMS/coolant flow control/min-max T ==
  T : Inport
  Coolant : Inport  Port=2
  Bus Creator1 : BusCreator  Inputs=3
  MinMax2 : MinMax
  MinMax3 : MinMax  Function=max
  plot T : Outport
  max T : Outport  Port=2
  wires:
  MinMax2/1 -> Bus Creator1/1  "min T"
  Bus Creator1/1 -> plot T/1  "Pack"
  MinMax3/1 -> max T/1, Bus Creator1/2  "max T"
  T/1 -> MinMax2/1, MinMax3/1
  Coolant/1 -> Bus Creator1/3  "coolant T"

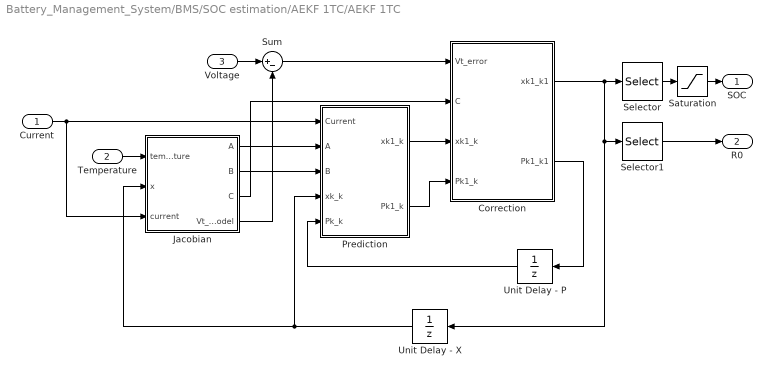
== system Battery_Management_System/BMS/SOC estimation/AEKF 1TC/AEKF 1TC ==
  Current : Inport
  Temperature : Inport  Port=2
  Voltage : Inport  Port=3
  Correction : Subsystem
  Jacobian : Subsystem
  Prediction : Subsystem
  Saturation : Saturate  UpperLimit=1  LowerLimit=0
  Selector : Selector  InputPortWidth=3  IndexOptions=Index vector (dialog)  Indices=1  OutputSizes=1
  Selector1 : Selector  InputPortWidth=3  IndexOptions=Index vector (dialog)  Indices=3  OutputSizes=1
  Sum : Sum  Inputs=|+-
  Unit Delay - P : UnitDelay  InitialCondition=P0  SampleTime=Ts  HasFrameUpgradeWarning=on
  Unit Delay - X : UnitDelay  InitialCondition=x0  SampleTime=Ts  HasFrameUpgradeWarning=on
  SOC : Outport  VectorParamsAs1DForOutWhenUnconnected=off
  R0 : Outport  Port=2  VectorParamsAs1DForOutWhenUnconnected=off
  wires:
  Prediction/1(xk1_k) -> Correction/3(xk1_k)
  Prediction/2(Pk1_k) -> Correction/4(Pk1_k)
  Correction/2(Pk1_k1) -> Unit Delay - P/1
  Unit Delay - P/1 -> Prediction/5(Pk_k)
  Unit Delay - X/1 -> Jacobian/2(x), Prediction/4(xk_k)
  Correction/1(xk1_k1) -> Selector/1, Selector1/1, Unit Delay - X/1
  Sum/1 -> Correction/1(Vt_error)
  Temperature/1 -> Jacobian/1(temperature)
  Jacobian/1(A) -> Prediction/2(A)
  Jacobian/2(B) -> Prediction/3(B)
  Jacobian/3(C) -> Correction/2(C)
  Voltage/1 -> Sum/1
  Jacobian/4(Vt_model) -> Sum/2
  Current/1 -> Prediction/1(Current), Jacobian/3(current)
  Selector/1 -> Saturation/1
  Saturation/1 -> SOC/1
  Selector1/1 -> R0/1

== system Battery_Management_System/BMS/coolant flow control/cooling system pump/FlwR_calc ==
  Max T : Inport
  Ambient : Inport  Port=2
  FlwR calc : Subsystem
  Step Change : Subsystem
  step : Constant  Value=.25  SampleTime=samplingTime
  output : Outport
  wires:
  FlwR calc/1(FlwR) -> Step Change/1(input)
  Max T/1 -> FlwR calc/1(Max T)
  step/1 -> Step Change/2(Step size)
  Ambient/1 -> FlwR calc/2(Ambient)
  Step Change/1(output) -> output/1

== system Battery_Management_System/BMS/coolant flow control/cooling system pump/pump power calc ==
  FlwR : Inport
  Power at max flow : Gain  Gain=500
  Saturation : Saturate  UpperLimit=500  LowerLimit=0
  Power : Outport
  wires:
  FlwR/1 -> Power at max flow/1
  Saturation/1 -> Power/1
  Power at max flow/1 -> Saturation/1

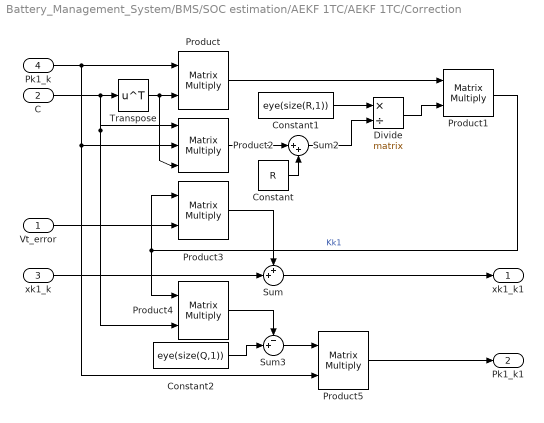
== system Battery_Management_System/BMS/SOC estimation/AEKF 1TC/AEKF 1TC/Correction ==
  Vt_error : Inport
  C : Inport  Port=2
  xk1_k : Inport  Port=3
  Pk1_k : Inport  Port=4
  Constant : Constant  Value=R
  Constant1 : Constant  Value=eye(size(R,1))
  Constant2 : Constant  Value=eye(size(Q,1))
  Divide : Product  Inputs=*/  Multiplication=Matrix(*)
  Product{,1,3..5} (5 alike) : Product  Multiplication=Matrix(*)
  Product2 : Product  Inputs=3  Multiplication=Matrix(*)
  Sum : Sum  Inputs=++|
  Sum2 : Sum  Inputs=|++
  Sum3 : Sum  Inputs=-+|
  Transpose : Math  Operator=transpose
  xk1_k1 : Outport
  Pk1_k1 : Outport  Port=2
  wires:
  C/1 -> Product4/2, Product2/1, Transpose/1
  Transpose/1 -> Product2/3, Product/2
  Pk1_k/1 -> Product5/2, Product2/2, Product/1
  Product/1 -> Product1/1
  Product2/1 -> Sum2/1
  Constant/1 -> Sum2/2
  Product1/1 -> Product4/1, Product3/1  "Kk1"
  Sum2/1 -> Divide/2
  Divide/1 -> Product1/2
  Constant1/1 -> Divide/1
  xk1_k/1 -> Sum/2
  Vt_error/1 -> Product3/2
  Product3/1 -> Sum/1
  Sum/1 -> xk1_k1/1
  Constant2/1 -> Sum3/2
  Product4/1 -> Sum3/1
  Sum3/1 -> Product5/1
  Product5/1 -> Pk1_k1/1

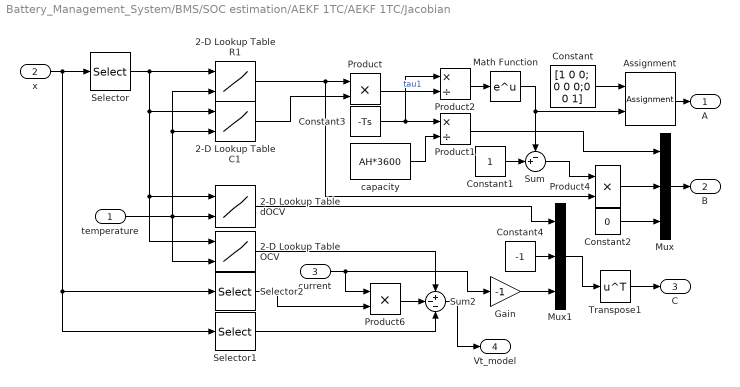
== system Battery_Management_System/BMS/SOC estimation/AEKF 1TC/AEKF 1TC/Jacobian ==
  temperature : Inport
  x : Inport  Port=2
  current : Inport  Port=3
  2-D Lookup Table C1 : Lookup_n-D  BreakpointsForDimension1=SOC_vec  BreakpointsForDimension2=T_vec  Table=C1_mat  InternalRulePriority=Speed  RndMeth=Simplest
      settings: InputPortMap=u0,u1
  2-D Lookup Table OCV : Lookup_n-D  BreakpointsForDimension1=SOC_vec  BreakpointsForDimension2=T_vec  Table=V0_mat  InternalRulePriority=Speed  RndMeth=Simplest
      settings: InputPortMap=u0,u1
  2-D Lookup Table R1 : Lookup_n-D  BreakpointsForDimension1=SOC_vec  BreakpointsForDimension2=T_vec  Table=R1_mat  InternalRulePriority=Speed  RndMeth=Simplest
      settings: InputPortMap=u0,u1
  2-D Lookup Table dOCV : Lookup_n-D  BreakpointsForDimension1=SOC_vec  BreakpointsForDimension2=T_vec  Table=dV0_mat  InternalRulePriority=Speed  RndMeth=Simplest
      settings: InputPortMap=u0,u1
  Assignment : Assignment  NumberOfDimensions=2  DiagnosticForDimensions=Warning  IndexOptions=Index vector (dialog),Index vector (dialog)  Indices=2,2  OutputSizes=1,1
  Constant : Constant  Value=|
      | [1 0 0;
      | 0 0 0;0 0 1]
  Constant1 : Constant
  Constant2 : Constant  Value=0
  Constant3 : Constant  Value=-Ts
  Constant4 : Constant  Value=-1
  Gain : Gain  Gain=-1
  Math Function : Math
  Mux : Mux  Inputs=3
  Mux1 : Mux  Inputs=3
  Product : Product
  Product1 : Product  Inputs=*/
  Product2 : Product  Inputs=*/
  Product4 : Product
  Product6 : Product
  Selector : Selector  InputPortWidth=3  IndexOptions=Index vector (dialog)  Indices=1  OutputSizes=1
  Selector1 : Selector  InputPortWidth=3  IndexOptions=Index vector (dialog)  Indices=2  OutputSizes=1
  Selector2 : Selector  InputPortWidth=3  IndexOptions=Index vector (dialog)  Indices=3  OutputSizes=1
  Sum : Sum  Inputs=-+|
  Sum2 : Sum  Inputs=+--
  Transpose1 : Math  Operator=transpose
  capacity : Constant  Value=AH*3600
  A : Outport
  B : Outport  Port=2
  C : Outport  Port=3
  Vt_model : Outport  Port=4
  wires:
  Constant2/1 -> Mux/3
  Gain/1 -> Mux1/3
  current/1 -> Product6/1, Gain/1
  temperature/1 -> 2-D Lookup Table R1/2, 2-D Lookup Table C1/2, 2-D Lookup Table dOCV/2, 2-D Lookup Table OCV/2
  Selector/1 -> 2-D Lookup Table OCV/1, 2-D Lookup Table dOCV/1, 2-D Lookup Table C1/1, 2-D Lookup Table R1/1
  x/1 -> Selector1/1, Selector2/1, Selector/1
  Constant/1 -> Assignment/1
  Math Function/1 -> Sum/1, Assignment/2
  2-D Lookup Table R1/1 -> Product4/2, Product/1
  2-D Lookup Table C1/1 -> Product/2
  Product/1 -> Product2/2  "tau1"
  Constant3/1 -> Product1/1, Product2/1
  Product2/1 -> Math Function/1
  Assignment/1 -> A/1
  Constant1/1 -> Sum/2
  Sum/1 -> Product4/1
  Product1/1 -> Mux/1
  Product4/1 -> Mux/2
  Mux/1 -> B/1
  Constant4/1 -> Mux1/2
  Product6/1 -> Sum2/2
  Selector1/1 -> Sum2/3
  Mux1/1 -> Transpose1/1
  Transpose1/1 -> C/1
  Sum2/1 -> Vt_model/1
  2-D Lookup Table OCV/1 -> Sum2/1
  2-D Lookup Table dOCV/1 -> Mux1/1
  Selector2/1 -> Product6/2
  capacity/1 -> Product1/2

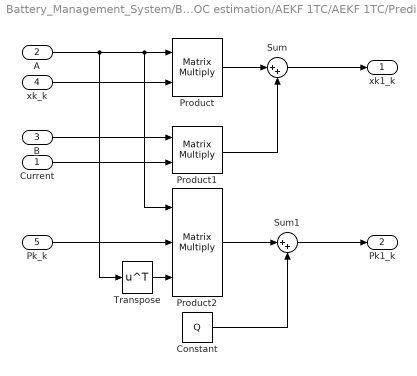
== system Battery_Management_System/BMS/SOC estimation/AEKF 1TC/AEKF 1TC/Prediction ==
  Current : Inport
  A : Inport  Port=2
  B : Inport  Port=3
  xk_k : Inport  Port=4
  Pk_k : Inport  Port=5
  Constant : Constant  Value=Q
  Product : Product  Multiplication=Matrix(*)
  Product1 : Product  Multiplication=Matrix(*)
  Product2 : Product  Inputs=3  Multiplication=Matrix(*)
  Sum : Sum  Inputs=|++
  Sum1 : Sum  Inputs=|++
  Transpose : Math  Operator=transpose
  xk1_k : Outport
  Pk1_k : Outport  Port=2
  wires:
  A/1 -> Transpose/1, Product2/1, Product/1
  xk_k/1 -> Product/2
  B/1 -> Product1/1
  Current/1 -> Product1/2
  Product/1 -> Sum/1
  Product1/1 -> Sum/2
  Sum/1 -> xk1_k/1
  Pk_k/1 -> Product2/2
  Transpose/1 -> Product2/3
  Product2/1 -> Sum1/1
  Constant/1 -> Sum1/2
  Sum1/1 -> Pk1_k/1

== system Battery_Management_System/BMS/coolant flow control/cooling system pump/FlwR_calc/FlwR calc ==
  Max T : Inport
  Ambient : Inport  Port=2
  Gain1 : Gain  Gain=.1
  Saturation : Saturate  UpperLimit=0.95  LowerLimit=0.001
  Subtract : Sum  Inputs=+-
  FlwR : Outport
  wires:
  Subtract/1 -> Gain1/1
  Ambient/1 -> Subtract/2
  Gain1/1 -> Saturation/1
  Saturation/1 -> FlwR/1
  Max T/1 -> Subtract/1

== system Battery_Management_System/BMS/coolant flow control/cooling system pump/FlwR_calc/Step Change ==
  input : Inport
  Step size : Inport  Port=2
  MinMax4 : MinMax  Function=max  Inputs=2
  Mod : Math  Operator=mod
  Subtract1 : Sum  Inputs=+-
  output : Outport
  wires:
  Mod/1 -> Subtract1/2
  MinMax4/1 -> output/1
  Subtract1/1 -> MinMax4/1
  input/1 -> Subtract1/1, Mod/1
  Step size/1 -> MinMax4/2, Mod/2

== matlab function Battery_Management_System/BMS/SOC estimation/SeriesStringData <Ns=20,Np=1> ==
  data: I input; Is output; T input; V input; Ts output; Vs output
function [Is,Ts,Vs] = seriesStr(I,T,V)
    Ns=20;
    Np=1;
    Is=zeros(Ns,1);
    Ts=zeros(Ns,1);
    Vs=zeros(Ns,1);
    for itr=1:Ns
        Is(itr,1)=-I/Np;
        Ts(itr,1)=T(itr,1);
        Vs(itr,1)=V(itr,1);
    end
end
